simulink model "modelo"  (Simulink 8.4)
settings: Solver=ode45  StartTime=0.0  StopTime=100  RelTol=1e-3
undefined symbols (not defined in the file): den, Kd, Ki, Kp, Mp, num, tp, tr, ts, ys
libraries: simulink_need_slupdate x1
settings Model: Creator=usuario_local  LastModifiedBy=usuario_local  ExtModeTrigMode=oneshot  ExtModeArmWhenConnect=off
settings DataIOCC: LimitDataPoints=off  SignalLoggingName=sigsOut
settings OptimizationCC: BooleanDataType=off  ExpressionDepthLimit=128
settings DebuggingCC: SaveWithParameterizedLinksMsg=none  SignalResolutionControl=TryResolveAllWithWarning  SolverPrmCheckMsg=none  MultiTaskDSMMsg=warning  MultiTaskCondExecSysMsg=none  FcnCallInpInsideContextMsg=EnableAllAsError  StateNameClashWarn=none
settings HardwareCC: TargetUnknown=on
settings RTWCC: IncludeERTFirstTime=on

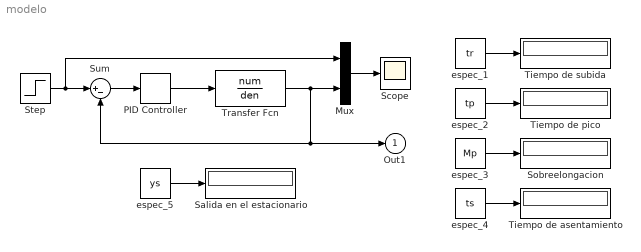
== system modelo ==
  Mux : Mux  Inputs=2
  PID Controller : simulink_need_slupdate/PID Controller  P=Kp  I=Ki  D=Kd
  Salida en el estacionario : Display
  Scope : Scope
      settings: TimeRange=100  YMin=0  YMax=1.4
  Sobreelongacion : Display
  Step : Step  Time=0  SampleTime=0.01
  Sum : Sum  Inputs=|+-  SaturateOnIntegerOverflow=on  InputSameDT=on  OutDataTypeStr=Inherit: Same as first input
  Tiempo de asentamiento : Display
  Tiempo de pico : Display
  Tiempo de subida : Display
  Transfer Fcn : TransferFcn  Numerator=num  Denominator=den
  espec_1 : Constant  Value=tr
  espec_2 : Constant  Value=tp
  espec_3 : Constant  Value=Mp
  espec_4 : Constant  Value=ts
  espec_5 : Constant  Value=ys
  Out1 : Outport
  wires:
  Sum/1 -> PID Controller/1
  Step/1 -> Sum/1, Mux/1
  Mux/1 -> Scope/1
  PID Controller/1 -> Transfer Fcn/1
  Transfer Fcn/1 -> Mux/2, Sum/2, Out1/1
  espec_1/1 -> Tiempo de subida/1
  espec_2/1 -> Tiempo de pico/1
  espec_3/1 -> Sobreelongacion/1
  espec_4/1 -> Tiempo de asentamiento/1
  espec_5/1 -> Salida en el estacionario/1
